simulink model "tesbackup"  (R2024a)
settings: Solver=VariableStepAuto  StartTime=0.0  StopTime=0.5  RelTol=1e-3
libraries: spsDistributedParametersLineLib x1, spsThreePhaseSeriesRLCLoadLib x1, spsThreePhaseVIMeasurementLib x1, spsThreePhaseFaultLib x1, spsThreePhaseSourceLib x1, sps_lib x1
settings Model: Creator=EE-106  LastModifiedBy=EE-106

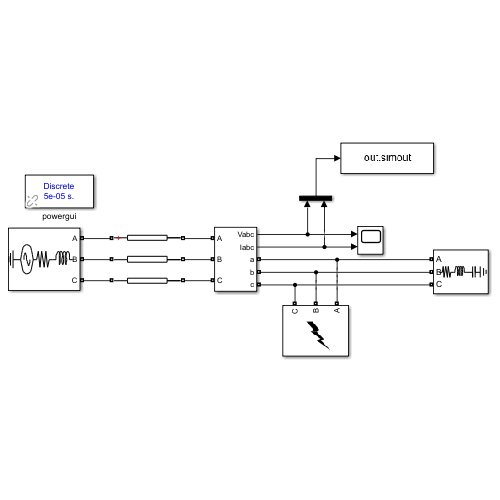
[thumbnail: Simulink's stored preview of the top-level diagram]
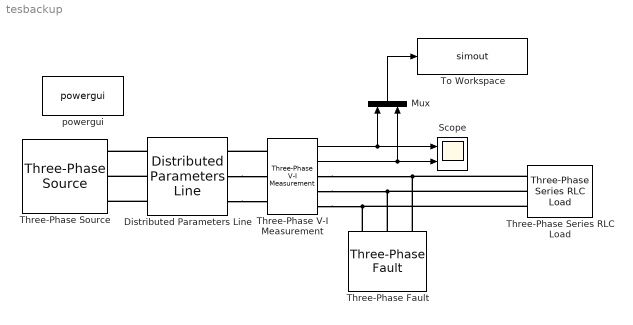
== system tesbackup ==
  Distributed Parameters Line : spsDistributedParametersLineLib/Distributed Parameters Line  Phases=3  Length=100  Frequency=60  Resistance=[0.01273 0.3864]  Inductance="[0.9337e-3  4.1264e-3]"  Capacitance=[12.74e-9 7.751e-9]  x1=[-0.0006 -6.54180057828466e-12 5914.63245859974 -23638.8078476183;-0.00055 -6.46347059825723e-12 6359.13638288504 -23523.126876349;-0.0005 -6.38284417790281e-12 6801.38093629327 -23399.0882501086;-0.00045 -6.29994996340464e-12 7241.20899144041 -23266.7360392305;-0.0004 -6.21481740668244e-12 7678.46427951277 -23126.1172678249;-0.00035 -6.12747675492822e-12 8112.99144578853 -22977.2818970718;-0.0003 -6.03795903985969e-12 8544.63610483456 -22820.2828074698;-0.00025 -5.94629606669475e-12 8973.24489535885 -22655.1757800477;-0.0002 -5.8525204028513e-12 9398.66553469898 -22482.0194765463;-0.00015 -5.75666536637618e-12 9820.74687292748 -22300.8754185756;-0.0001 -5.65876501410743e-12 10239.3389465547 -22111.8079657569;-5e-05 -5.55885412957405e-12 10654.29303181 -21914.884292856]  x2=[-0.0006 9.32220968025092e-12 -2090.23125560322 -22808.3970568346;-0.00055 9.32141111933284e-12 -1659.95723406626 -22843.7427972123;-0.0005 9.31730070542905e-12 -1229.09343762812 -22870.9722645475;-0.00045 9.30987989895005e-12 -797.792950144069 -22890.0757843398;-0.0004 9.29915133647305e-12 -366.209010623616 -22901.0465691998;-0.00035 9.2851188298052e-12 65.5050412145663 -22903.8807212598;-0.0003 9.26778736462931e-12 497.195819423514 -22898.577233559;-0.00025 9.24716309873243e-12 928.709946325278 -22885.1379904015;-0.0002 9.22325335981803e-12 1359.89410700527 -22863.5677666862;-0.00015 9.1960666429025e-12 1790.59510378435 -22833.874226211;-0.0001 9.1656126072969e-12 2220.65991064917 -22796.0679189494;-5e-05 9.13190207317508e-12 2649.93572762168 -22750.1622773024]  x3=[-0.0006 -1.65204104133637e-14 31.482698286299 139.643186193758;-0.00055 -1.40012996122372e-14 28.8450492832622 140.211778654922;-0.0005 -1.14772142160273e-14 26.1971517715641 140.730554538765;-0.00045 -8.94905102025656e-15 23.5399465365825 141.199329526685;-0.0004 -6.41770826927029e-15 20.8743776706846 141.617937065162;-0.00035 -3.88408533709462e-15 18.2013922377961 141.98622842493;-0.0003 -1.34908240789321e-15 15.5219399369136 142.304072753823;-0.00025 1.18639984386391e-15 12.8369727646811 142.571357123264;-0.0002 3.72146057340569e-15 10.1474446771501 142.78798656839;-0.00015 6.2551990857259e-15 7.45431125084349 142.95388412179;-0.0001 8.78671515559583e-15 4.75852934324407 143.068990840853;-5e-05 1.131510934741e-14 2.06105675282729 143.13326582871]  x4=[-0.0006 -5.5315410957477e-14 -28.5491669252259 -311.525690340176;-0.00055 -5.77538095203255e-14 -22.6723220395141 -312.008455794685;-0.0005 -6.0171688429653e-14 -16.7874217857385 -312.380366130516;-0.00045 -6.25681886245961e-14 -10.8965570409377 -312.641289209696;-0.0004 -6.49424586400466e-14 -5.00182080130561 -312.791132327499;-0.00035 -6.72936549091735e-14 0.894692561440513 -312.829842245378;-0.0003 -6.96209420631379e-14 6.79088804417972 -312.757405209883;-0.00025 -7.19234932278956e-14 12.6846707567324 -312.573846957548;-0.0002 -7.42004903179816e-14 18.5739466661649 -312.279232705747;-0.00015 -7.6451124327172e-14 24.4566233407888 -311.873667129519;-0.0001 -7.867459561592e-14 30.3306106935929 -311.357294324384;-5e-05 -8.08701141954641e-14 36.1938217248403 -310.73029775514]  x5=0.000565541566995742  V1=[1.627e-11 2.437e+04 2.437e+04;377 377 377;-2.891 0.3413 -1.229]  V2=[1.741e-11 2.29e+04 2.29e+04;377 377 377;0.7768 0.004784 -1.566]  I1=[1.489e-13 143.1 143.1;377 377 377;-0.8046 3.016 1.445]  I2=[1.882e-13 312.8 312.8;377 377 377;2.3 0.004784 -1.566]  nHarmo=1  Measurements=None  Decoupling=off  VsMag0=0  VrMag0=0  VsAngle0=0  VrAngle0=0  IsMag0=0  IrMag0=0  IsAngle0=0  IrAngle0=0
      settings: LibrarySourceBlock=sps_lib/Power Grid Elements/Distributed Parameters Line
  Mux : Mux  Inputs=2
  Scope : Scope  NumInputPorts=2
  Three-Phase Series RLC Load : spsThreePhaseSeriesRLCLoadLib/Three-Phase Series RLC Load  LConnTagsString=A|B|C  Configuration=Y (grounded)  NominalVoltage=1000  Vabc=[1e3 1e3 1e3]  Vabcp=[1e3 1e3 1e3]  NominalFrequency=60  UnbalancedPower=off  ActivePower=10e3  InductivePower=100  CapacitivePower=100  Pabc=[10e3 9e3 11e3]  QLabc=[100 90 110]  QCabc=[100 90 110]  Pabcp=[10e3 9e3 11e3]  QLabcp=[100 90 110]  QCabcp=[100 90 110]  Measurements=None  LoadType=constant Z
  Three-Phase V-I Measurement : spsThreePhaseVIMeasurementLib/Three-Phase V-I Measurement  VoltageMeasurement=phase-to-ground  SetLabelV=off  LabelV=Vabc  Vpu=on  VpuLL=off  CurrentMeasurement=yes  SetLabelI=off  LabelI=Iabc  Ipu=on  Pbase=500e3  Vbase=100e6  OutputType=Complex  PhasorSimulation=off  PSBequivalent=0
  Three-Phase Fault : spsThreePhaseFaultLib/Three-Phase Fault  InitialStates=0  FaultA=on  FaultB=on  FaultC=off  GroundFault=on  SwitchTimes="[10/60  20/60]"  External=off  SwitchStatus=NaN  FaultResistance=0.0001  GroundResistance=0.01  SnubberResistance=1e6  SnubberCapacitance=inf  Measurements=None
  Three-Phase Source : spsThreePhaseSourceLib/Three-Phase Source  InternalConnection=Yg  VoltagePhases=off  Voltage=25e3  PhaseAngle=0  Voltage_phases=[25e3 25e3 25e3]/sqrt(3)  PhaseAngles_phases=[0 -120 +120]  Frequency=60  NonIdealSource=on  SpecifyImpedance=off  Resistance=0.8929  Inductance=16.58e-3  ShortCircuitLevel=100e6  BaseVoltage=25e3  XRratio=7  BusType=PV  Pref=10e3  Qref=0  Prefabc=[10e3, 10e3, 10e3]  Qrefabc=[0, 0, 0]  Qmin=-inf  Qmax=inf
  To Workspace : ToWorkspace  VariableName=simout  SaveFormat=Timeseries  SampleTime=-1
  powergui : sps_lib/powergui  Priority=1  SimulationMode=Discrete  SampleTime=5e-05  frequency=60  Iterations=50  frequencyindice=60  Pbase=100e6  ErrMax=1e-4  UnitsV=kV  UnitsW=MW  buscounter=0  FunctionMessages=off  echomessages=off  EnableUseOfTLC=off  CurrentSourceSwitches=off  DisableSnubberDevices=off  DisableRonSwitches=off  DisableVfSwitches=off  DisplayEquations=off  AutomaticDiscreteSolvers=off  SolverType=Tustin/Backward Euler (TBE)  Interpol=off  ExternalGateDelay=off  methode=off  Ts=100  x0status=blocks  SPID=on  SwTol=0  HookPort=off  NonlinearTolerance=1e-4  nMaxIteration=100  ContinueOnMaxIteration=off  RestoreLinks=warning  ResistiveCurrentMeasurement=off  Frange=[0:2:500]  Ylog=off  Xlog=on  ShowGrid=off  save=off  variable=ZData  structure=0  ZoomFFT=off  StartTime=0.0  cycles=1  DisplayStyle=1  fundamental=60  FreqAxis=off  MaxFrequency=1000  frequencyindicesteady=1  RmsSteady=1  display=off
  wires:
  Three-Phase V-I Measurement/1 -> Mux/1, Scope/1
  Three-Phase V-I Measurement/2 -> Mux/2, Scope/2
  Mux/1 -> To Workspace/1
  connections:
  Distributed Parameters Line/LConn1 -- Three-Phase Source/RConn1
  Distributed Parameters Line/LConn2 -- Three-Phase Source/RConn2
  Distributed Parameters Line/LConn3 -- Three-Phase Source/RConn3
  Three-Phase V-I Measurement/LConn1 -- Distributed Parameters Line/RConn1
  Distributed Parameters Line/RConn2 -- Three-Phase V-I Measurement/LConn2
  Distributed Parameters Line/RConn3 -- Three-Phase V-I Measurement/LConn3
  Three-Phase V-I Measurement/RConn1 -- Three-Phase Series RLC Load/LConn1 -- Three-Phase Fault/LConn1
  Three-Phase V-I Measurement/RConn2 -- Three-Phase Fault/LConn2 -- Three-Phase Series RLC Load/LConn2
  Three-Phase V-I Measurement/RConn3 -- Three-Phase Series RLC Load/LConn3 -- Three-Phase Fault/LConn3
